simulink subsystem "SimpleRXNoiseModel"  (R2021a)
settings: Solver=VariableStepAuto  StartTime=0.0  StopTime=10.0  RelTol=1e-3
undefined symbols (not defined in the file or in its folder): G_bpf_rx, G_hpa_rx, G_lna_rx, G_lpf_rx, G_mix_rx, N_ant_rx, N_bpf_rx, N_hpa_rx, N_lna_rx, N_lpf_rx, N_mix_rx
libraries: simulink x6
settings Model: Creator=drewd  LastModifiedBy=drewd

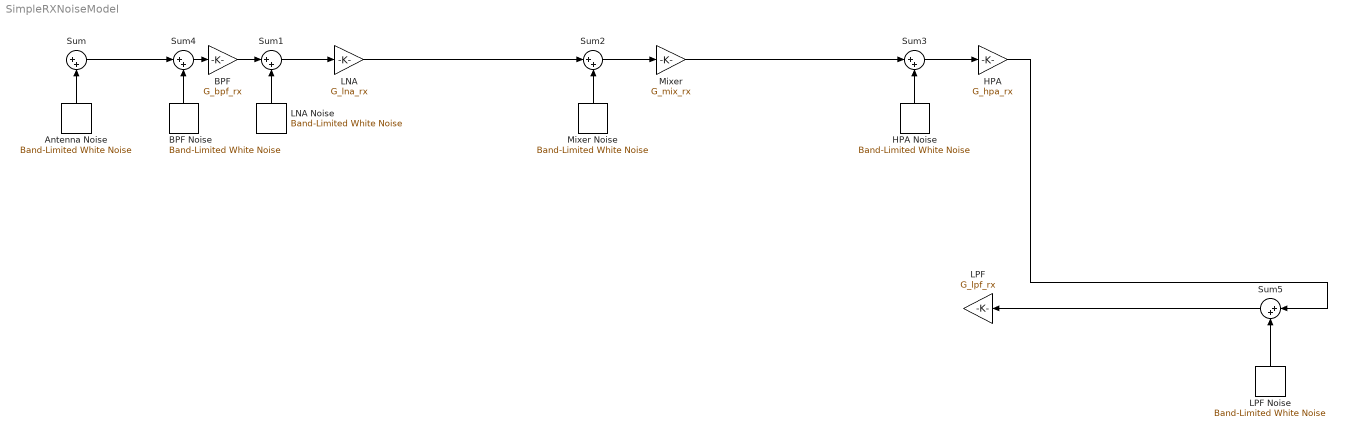
== system SimpleRXNoiseModel ==
  Antenna Noise : simulink/Sources/Band-Limited White Noise  Cov=[N_ant_rx]  Ts=0.1  seed=[23341]
  BPF : Gain  Gain=G_bpf_rx
  BPF Noise : simulink/Sources/Band-Limited White Noise  Cov=[N_bpf_rx]  Ts=0.1  seed=[23341]
  HPA : Gain  Gain=G_hpa_rx
  HPA Noise : simulink/Sources/Band-Limited White Noise  Cov=[N_hpa_rx]  Ts=0.1  seed=[23341]
  LNA : Gain  Gain=G_lna_rx
  LNA Noise : simulink/Sources/Band-Limited White Noise  Cov=[N_lna_rx]  Ts=0.1  seed=[23341]
  LPF : Gain  Gain=G_lpf_rx
  LPF Noise : simulink/Sources/Band-Limited White Noise  Cov=[N_lpf_rx]  Ts=0.1  seed=[23341]
  Mixer : Gain  Gain=G_mix_rx
  Mixer Noise : simulink/Sources/Band-Limited White Noise  Cov=[N_mix_rx]  Ts=0.1  seed=[23341]
  Sum{,1..5} (6 alike) : Sum  Inputs=|++
  wires:
  Antenna Noise/1 -> Sum/2
  LNA Noise/1 -> Sum1/2
  Sum1/1 -> LNA/1
  Sum2/1 -> Mixer/1
  Mixer Noise/1 -> Sum2/2
  LNA/1 -> Sum2/1
  Mixer/1 -> Sum3/1
  HPA Noise/1 -> Sum3/2
  Sum3/1 -> HPA/1
  BPF/1 -> Sum1/1
  Sum4/1 -> BPF/1
  BPF Noise/1 -> Sum4/2
  Sum/1 -> Sum4/1
  Sum5/1 -> LPF/1
  LPF Noise/1 -> Sum5/2
  HPA/1 -> Sum5/1
  ? -> Sum/1
